simulink model "RL_tcp_2021b"  (R2021b)
settings: Solver=VariableStepAuto  StartTime=0.0  StopTime=inf  RelTol=1e-3
undefined symbols (not defined in the file or in its folder): A, alpha_b_gain, B, C, Discrete, fitresultpowertwoFL, fitresultpowertwoFR, fitresultpowertwoRL, fitresultpowertwoRR, R, rotateCorrectionCoef, Tf, Time, Ts, VRef, x_norm_min, y_norm_min, y_norm_range, z_l_gain
libraries: svdutilitieslib x15, simulink x9, ctrlSharedLib x3, instrumentlib x2, deeplib x2, aerolibanimutils x1
settings Model: Creator=4DLab5  LastModifiedBy=n7729

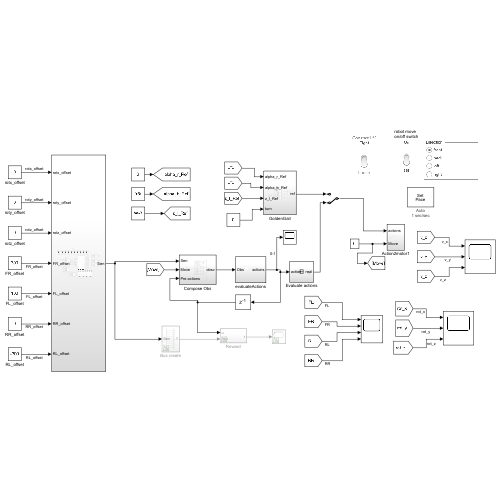
[thumbnail: Simulink's stored preview of the top-level diagram]
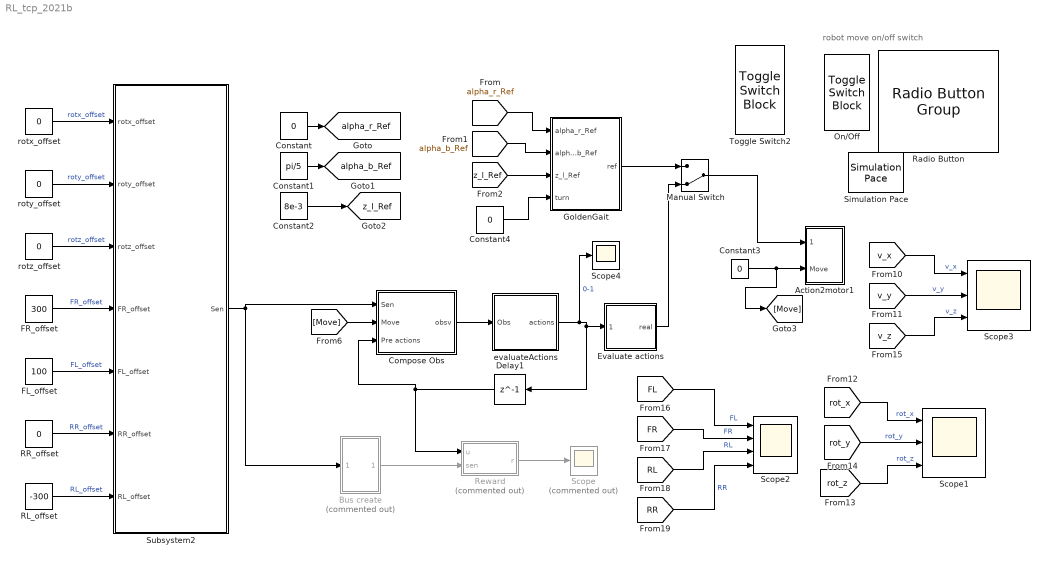
== system RL_tcp_2021b ==
  note: robot move
      | on/off switch
  Action2motor1 : Subsystem
  Bus create : Subsystem  Commented=on
  Compose Obs : Subsystem
  Constant : Constant  Value=0
  Constant1 : Constant  Value=pi/5
  Constant2 : Constant  Value=8e-3
  Constant3 : Constant  Value=0
  Constant4 : Constant  Value=0
  Delay1 : Delay  DelayLength=1  InitialCondition=[0.5;0.5;0.5;0.5]  SampleTime=0.05
  Evaluate actions : Subsystem
  FL_offset : Constant  Value=100
  FR_offset : Constant  Value=300
  GoldenGait : Subsystem
  Manual Switch : ManualSwitch  CurrentSetting=0
  On/Off : ToggleSwitchBlock  LabelPosition=Hide
      settings: Values={{'Off', 'On'}, [0 1]}
  RL_offset : Constant  Value=-300
  RR_offset : Constant  Value=0
  Radio Button : RadioButtonGroup  LabelPosition=Hide  SelectedLabel=front  ButtonGroupName=Direction
      settings: Values={{'front', 'back', 'left', 'right'}, [0 3.1416 1.5708 -1.5708]}
  Reward : Subsystem  Commented=on
  Scope : Scope  Commented=on
  Scope1 : Scope  NumInputPorts=3
  Scope2 : Scope  NumInputPorts=4
  Scope3 : Scope  NumInputPorts=3
  Scope4 : Scope
  Simulation Pace : aerolibanimutils/Simulation Pace  SimulationPace=1  SleepMode=Auto  OutputPaceError=off  SampleTime=0.05
  Subsystem2 : Subsystem
  Toggle Switch2 : ToggleSwitchBlock
      settings: Values={{'Loose', 'Tight'}, [0 1]}
  evaluateActions : Subsystem
  rotx_offset : Constant  Value=0
  roty_offset : Constant  Value=0
  rotz_offset : Constant  Value=0
  tag scope: alpha_b_Ref=global, alpha_r_Ref=global, z_l_Ref=global
  wires:
  RR_offset/1 -> Subsystem2/6(RR_offset)  "RR_offset"
  [v_x] -> Scope3/1  "v_x"
  RL_offset/1 -> Subsystem2/7(RL_offset)  "RL_offset"
  [Move] -> Compose Obs/2(Move)
  [rot_y] -> Scope1/2  "rot_y"
  Evaluate actions/1(real) -> Manual Switch/2
  FR_offset/1 -> Subsystem2/4(FR_offset)  "FR_offset"
  [RL] -> Scope2/3  "RL"
  [rot_z] -> Scope1/3  "rot_z"
  Constant4/1 -> GoldenGait/4(turn)
  [RR] -> Scope2/4  "RR"
  [alpha_r_Ref] -> GoldenGait/1(alpha_r_Ref)
  Delay1/1 -> Compose Obs/3(Pre actions), Reward/1(u)
  [z_l_Ref] -> GoldenGait/3(z_l_Ref)
  [v_z] -> Scope3/3  "v_z"
  [v_y] -> Scope3/2  "v_y"
  [FR] -> Scope2/2  "FR"
  [alpha_b_Ref] -> GoldenGait/2(alpha_b_Ref)
  [rot_x] -> Scope1/1  "rot_x"
  Manual Switch/1 -> Action2motor1/1(actions)
  [FL] -> Scope2/1  "FL"
  Subsystem2/1(Sen) -> Compose Obs/1(Sen), Bus create/1(Sen)
  Compose Obs/1(obsv) -> evaluateActions/1(Obs)
  Constant1/1 -> [alpha_b_Ref]
  Constant2/1 -> [z_l_Ref]
  Constant3/1 -> [Move], Action2motor1/2(Move)
  rotz_offset/1 -> Subsystem2/3(rotz_offset)  "rotz_offset"
  roty_offset/1 -> Subsystem2/2(roty_offset)  "roty_offset"
  Reward/1(r) -> Scope/1
  Constant/1 -> [alpha_r_Ref]
  Bus create/1(Outport) -> Reward/2(sen)
  FL_offset/1 -> Subsystem2/5(FL_offset)  "FL_offset"
  evaluateActions/1(actions) -> Scope4/1, Evaluate actions/1(action), Delay1/1  "0-1"
  GoldenGait/1(ref) -> Manual Switch/1
  rotx_offset/1 -> Subsystem2/1(rotx_offset)  "rotx_offset"

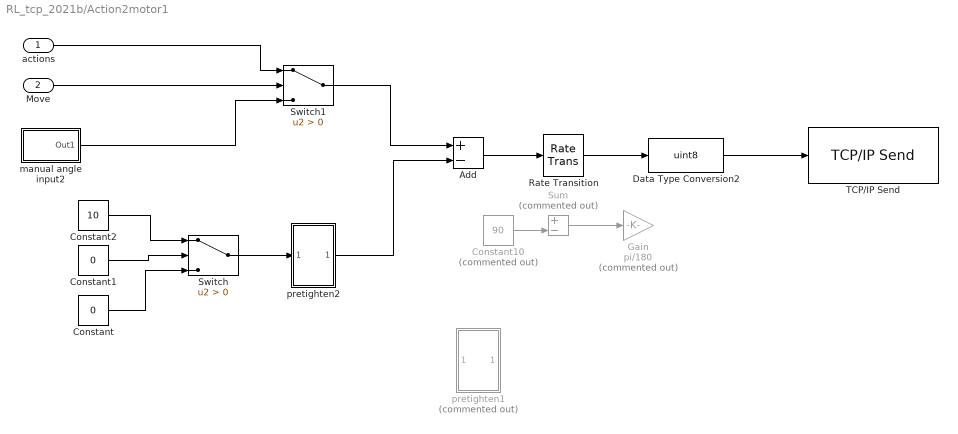
== system RL_tcp_2021b/Action2motor1 ==
  actions : Inport
  Move : Inport  Port=2
  Add : Sum  Inputs=+-
  Constant : Constant  Value=0
  Constant1 : Constant  Value=0
  Constant10 : Constant  Commented=on  Value=90
  Constant2 : Constant  Value=10
  Data Type Conversion2 : DataTypeConversion  OutDataTypeStr=uint8
  Gain : Gain  Commented=on  Gain=pi/180
  Rate Transition : RateTransition  OutPortSampleTime=0.05
  Sum : Sum  Commented=on  Inputs=+-
  Switch : Switch  Criteria=u2 > Threshold
  Switch1 : Switch  Criteria=u2 > Threshold
  TCP/IP Send : instrumentlib/TCP//IP Send  Priority=1  Host=192.168.0.103  Port=6666  ByteOrder=big-endian  EnableBlockingMode=on  Timeout=1  TransferDelay=on  SimulateUsing=Interpreted execution
  manual angle input2 : Subsystem
  pretighten1 : Subsystem  Commented=on
  pretighten2 : Subsystem
  wires:
  manual angle input2/1(Out1) -> Switch1/3
  pretighten2/1(Out1) -> Add/2
  Switch1/1 -> Add/1
  Switch/1 -> pretighten2/1(In1)
  Constant/1 -> Switch/3
  Constant2/1 -> Switch/1
  Data Type Conversion2/1 -> TCP/IP Send/1
  Add/1 -> Rate Transition/1
  Constant1/1 -> Switch/2
  Move/1 -> Switch1/2
  actions/1 -> Switch1/1
  Constant10/1 -> Sum/2
  Sum/1 -> Gain/1
  Rate Transition/1 -> Data Type Conversion2/1

== system RL_tcp_2021b/Bus create ==
  Sen : Inport
  Bus Creator : BusCreator  Inputs=10
  Demux : Demux  Outputs=10
  Outport : Outport
  wires:
  Sen/1 -> Demux/1
  Demux/1 -> Bus Creator/1  "rot_x"
  Demux/2 -> Bus Creator/2  "rot_y"
  Demux/3 -> Bus Creator/3  "rot_z"
  Bus Creator/1 -> Outport/1
  Demux/4 -> Bus Creator/4  "v_x"
  Demux/5 -> Bus Creator/5  "v_y"
  Demux/6 -> Bus Creator/6  "v_z"
  Demux/7 -> Bus Creator/7  "FnFR"
  Demux/8 -> Bus Creator/8  "FnFL"
  Demux/9 -> Bus Creator/9  "FnRL"
  Demux/10 -> Bus Creator/10  "FnRR"

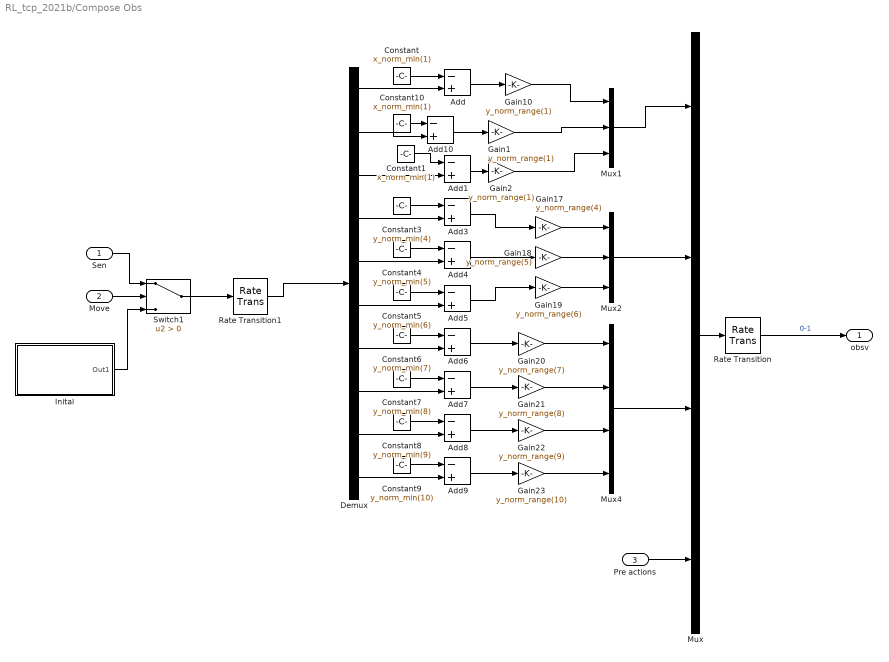
== system RL_tcp_2021b/Compose Obs ==
  Sen : Inport
  Move : Inport  Port=2
  Pre actions : Inport  Port=3
  Add{,1,3..10} (10 alike) : Sum  Inputs=-+
  Constant : Constant  Value=x_norm_min(1)
  Constant1 : Constant  Value=x_norm_min(1)
  Constant10 : Constant  Value=x_norm_min(1)
  Constant3 : Constant  Value=y_norm_min(4)
  Constant4 : Constant  Value=y_norm_min(5)
  Constant5 : Constant  Value=y_norm_min(6)
  Constant6 : Constant  Value=y_norm_min(7)
  Constant7 : Constant  Value=y_norm_min(8)
  Constant8 : Constant  Value=y_norm_min(9)
  Constant9 : Constant  Value=y_norm_min(10)
  Demux : Demux  Outputs=10
  Gain1 : Gain  Gain=y_norm_range(1)
  Gain10 : Gain  Gain=y_norm_range(1)
  Gain17 : Gain  Gain=y_norm_range(4)
  Gain18 : Gain  Gain=y_norm_range(5)
  Gain19 : Gain  Gain=y_norm_range(6)
  Gain2 : Gain  Gain=y_norm_range(1)
  Gain20 : Gain  Gain=y_norm_range(7)
  Gain21 : Gain  Gain=y_norm_range(8)
  Gain22 : Gain  Gain=y_norm_range(9)
  Gain23 : Gain  Gain=y_norm_range(10)
  Inital : Subsystem
  Mux : Mux
  Mux1 : Mux  Inputs=3
  Mux2 : Mux  Inputs=3
  Mux4 : Mux
  Rate Transition : RateTransition  OutPortSampleTime=Ts
  Rate Transition1 : RateTransition  OutPortSampleTime=Ts
  Switch1 : Switch  Criteria=u2 > Threshold
  obsv : Outport  VectorParamsAs1DForOutWhenUnconnected=off
  wires:
  Gain18/1 -> Mux2/2
  Gain19/1 -> Mux2/3
  Constant/1 -> Add/1
  Gain10/1 -> Mux1/1
  Add/1 -> Gain10/1
  Mux2/1 -> Mux/2
  Constant5/1 -> Add5/1
  Demux/1 -> Add/2
  Gain21/1 -> Mux4/2
  Demux/9 -> Add8/2
  Add9/1 -> Gain23/1
  Constant9/1 -> Add9/1
  Rate Transition/1 -> obsv/1  "0-1"
  Add3/1 -> Gain17/1
  Constant7/1 -> Add7/1
  Gain20/1 -> Mux4/1
  Gain17/1 -> Mux2/1
  Constant6/1 -> Add6/1
  Demux/4 -> Add3/2
  Mux4/1 -> Mux/3
  Mux/1 -> Rate Transition/1
  Add7/1 -> Gain21/1
  Mux1/1 -> Mux/1
  Demux/7 -> Add6/2
  Gain23/1 -> Mux4/4
  Demux/5 -> Add4/2
  Gain22/1 -> Mux4/3
  Constant4/1 -> Add4/1
  Constant3/1 -> Add3/1
  Constant8/1 -> Add8/1
  Add5/1 -> Gain19/1
  Add4/1 -> Gain18/1
  Add6/1 -> Gain20/1
  Add8/1 -> Gain22/1
  Demux/8 -> Add7/2
  Pre actions/1 -> Mux/4
  Demux/10 -> Add9/2
  Demux/6 -> Add5/2
  Move/1 -> Switch1/2
  Sen/1 -> Switch1/1
  Switch1/1 -> Rate Transition1/1
  Inital/1(Out1) -> Switch1/3
  Rate Transition1/1 -> Demux/1
  Demux/2 -> Add10/2
  Add10/1 -> Gain1/1
  Gain1/1 -> Mux1/2
  Constant10/1 -> Add10/1
  Add1/1 -> Gain2/1
  Demux/3 -> Add1/2
  Gain2/1 -> Mux1/3
  Constant1/1 -> Add1/1

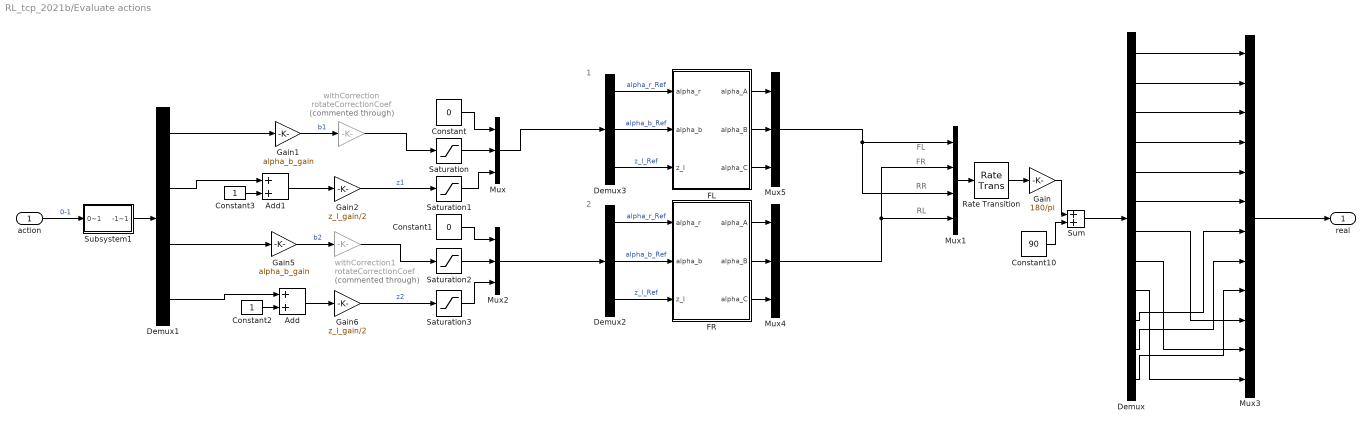
== system RL_tcp_2021b/Evaluate actions ==
  note: RL
  note: FR
  note: FL
  note: RR
  note: 2
  note: 1
  action : Inport
  Add : Sum
  Add1 : Sum
  Constant : Constant  Value=0
  Constant1 : Constant  Value=0
  Constant10 : Constant  Value=90
  Constant2 : Constant
  Constant3 : Constant
  Demux : Demux  Outputs=12
  Demux1 : Demux
  Demux2 : Demux  Outputs=3
  Demux3 : Demux  Outputs=3
  FL : MATLAB Function  TreatAsAtomicUnit=on
  FR : MATLAB Function  TreatAsAtomicUnit=on
  Gain : Gain  Gain=180/pi
  Gain1 : Gain  Gain=alpha_b_gain
  Gain2 : Gain  Gain=z_l_gain/2
  Gain5 : Gain  Gain=alpha_b_gain
  Gain6 : Gain  Gain=z_l_gain/2
  Mux{,2,4..5} (4 alike) : Mux  Inputs=3
  Mux1 : Mux
  Mux3 : Mux  Inputs=12
  Rate Transition : RateTransition  OutPortSampleTime=0.05
  Saturation : Saturate  UpperLimit=pi/5  LowerLimit=-pi/5
  Saturation1 : Saturate  UpperLimit=10e-3  LowerLimit=-10e-3
  Saturation2 : Saturate  UpperLimit=pi/5  LowerLimit=-pi/5
  Saturation3 : Saturate  UpperLimit=10e-3  LowerLimit=-10e-3
  Subsystem1 : Subsystem
  Sum : Sum
  withCorrection : Gain  Commented=through  Gain=rotateCorrectionCoef
  withCorrection1 : Gain  Commented=through  Gain=rotateCorrectionCoef
  real : Outport
  wires:
  Mux1/1 -> Rate Transition/1
  Constant/1 -> Mux/1
  withCorrection/1 -> Saturation/1
  Constant1/1 -> Mux2/1
  withCorrection1/1 -> Saturation2/1
  Mux2/1 -> Demux2/1
  Saturation/1 -> Mux/2
  Saturation2/1 -> Mux2/2
  Saturation1/1 -> Mux/3
  Saturation3/1 -> Mux2/3
  action/1 -> Subsystem1/1(0~1)  "0-1"
  Demux1/1 -> Gain1/1
  Gain1/1 -> withCorrection/1  "b1"
  Gain5/1 -> withCorrection1/1  "b2"
  Gain2/1 -> Saturation1/1  "z1"
  Gain6/1 -> Saturation3/1  "z2"
  Demux1/2 -> Add1/1
  Add1/1 -> Gain2/1
  Add/1 -> Gain6/1
  Constant2/1 -> Add/2
  Demux1/3 -> Gain5/1
  Constant3/1 -> Add1/2
  Demux1/4 -> Add/1
  Subsystem1/1(-1~1) -> Demux1/1
  Sum/1 -> Demux/1
  Demux/11 -> Mux3/8
  Gain/1 -> Sum/1
  Demux/2 -> Mux3/2
  Demux/10 -> Mux3/7
  Demux/9 -> Mux3/12
  Demux/5 -> Mux3/5
  Demux/1 -> Mux3/1
  Demux/7 -> Mux3/10
  Demux/8 -> Mux3/11
  Demux/4 -> Mux3/4
  Demux/12 -> Mux3/9
  Constant10/1 -> Sum/2
  Demux/6 -> Mux3/6
  Demux/3 -> Mux3/3
  Demux2/1 -> FR/1(alpha_r)  "alpha_r_Ref"
  FR/3(alpha_C) -> Mux4/3
  Demux2/2 -> FR/2(alpha_b)  "alpha_b_Ref"
  FR/2(alpha_B) -> Mux4/2
  FR/1(alpha_A) -> Mux4/1
  Mux4/1 -> Mux1/2, Mux1/4
  Demux2/3 -> FR/3(z_l)  "z_l_Ref"
  Mux3/1 -> real/1
  FL/1(alpha_A) -> Mux5/1
  Mux5/1 -> Mux1/3, Mux1/1
  Demux3/3 -> FL/3(z_l)  "z_l_Ref"
  FL/3(alpha_C) -> Mux5/3
  FL/2(alpha_B) -> Mux5/2
  Mux/1 -> Demux3/1
  Demux3/1 -> FL/1(alpha_r)  "alpha_r_Ref"
  Demux3/2 -> FL/2(alpha_b)  "alpha_b_Ref"
  Rate Transition/1 -> Gain/1

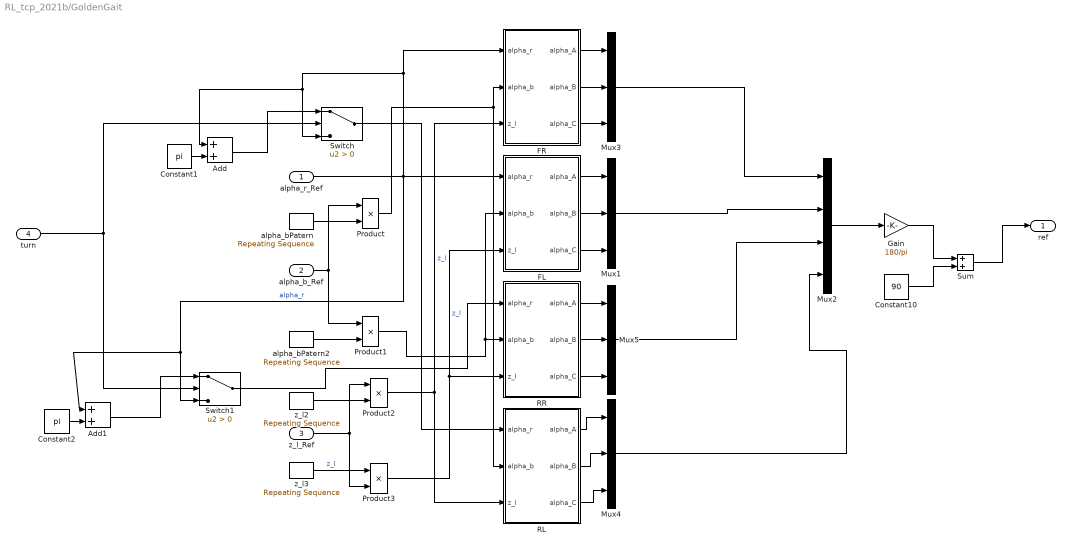
== system RL_tcp_2021b/GoldenGait ==
  alpha_r_Ref : Inport
  alpha_b_Ref : Inport  Port=2
  z_l_Ref : Inport  Port=3
  turn : Inport  Port=4
  Add : Sum
  Add1 : Sum
  Constant1 : Constant  Value=pi
  Constant10 : Constant  Value=90
  Constant2 : Constant  Value=pi
  FL : MATLAB Function  TreatAsAtomicUnit=on
  FR : MATLAB Function  TreatAsAtomicUnit=on
  Gain : Gain  Gain=180/pi
  Mux{1,3..5} (4 alike) : Mux  Inputs=3
  Mux2 : Mux
  Product{,1..3} (4 alike) : Product
  RL : MATLAB Function  TreatAsAtomicUnit=on
  RR : MATLAB Function  TreatAsAtomicUnit=on
  Sum : Sum
  Switch : Switch  Criteria=u2 > Threshold
  Switch1 : Switch  Criteria=u2 > Threshold
  alpha_bPatern : simulink/Sources/Repeating Sequence  rep_seq_t=[0 0.2 0.4 0.6 0.8]  rep_seq_y=[0 1 0 -1 0]
  alpha_bPatern2 : simulink/Sources/Repeating Sequence  rep_seq_t=[0 0.2 0.4 0.6 0.8]  rep_seq_y=[0 -1 0 1 0]
  z_l2 : simulink/Sources/Repeating Sequence  rep_seq_t=[0 0.2 0.4 0.6 0.8]  rep_seq_y=[0 1 1 1 0]
  z_l3 : simulink/Sources/Repeating Sequence  rep_seq_t=[0 0.2 0.4 0.6 0.8]  rep_seq_y=[1 1 0 1 1]
  ref : Outport
  wires:
  FR/1(alpha_A) -> Mux3/1
  Product2/1 -> FR/3(z_l), RL/3(z_l)  "z_l"
  FR/2(alpha_B) -> Mux3/2
  FR/3(alpha_C) -> Mux3/3
  Product3/1 -> FL/3(z_l), RR/3(z_l)  "z_l"
  FL/3(alpha_C) -> Mux1/3
  alpha_r_Ref/1 -> Switch1/3, Add1/1, FL/1(alpha_r), FR/1(alpha_r), Switch/3, Add/1  "alpha_r"
  FL/2(alpha_B) -> Mux1/2
  FL/1(alpha_A) -> Mux1/1
  alpha_bPatern/1 -> Product/2
  alpha_b_Ref/1 -> Product/1, Product1/1
  Product/1 -> RL/2(alpha_b), FR/2(alpha_b)
  alpha_bPatern2/1 -> Product1/2
  Product1/1 -> FL/2(alpha_b), RR/2(alpha_b)
  z_l2/1 -> Product2/2
  z_l_Ref/1 -> Product3/2, Product2/1
  z_l3/1 -> Product3/1  "z_l"
  RL/3(alpha_C) -> Mux4/3
  RL/2(alpha_B) -> Mux4/2
  RL/1(alpha_A) -> Mux4/1
  Mux3/1 -> Mux2/1
  RR/3(alpha_C) -> Mux5/3
  RR/1(alpha_A) -> Mux5/1
  RR/2(alpha_B) -> Mux5/2
  Switch/1 -> RL/1(alpha_r)
  Constant1/1 -> Add/2
  Add/1 -> Switch/1
  Switch1/1 -> RR/1(alpha_r)
  Add1/1 -> Switch1/1
  Constant2/1 -> Add1/2
  turn/1 -> Switch1/2, Switch/2
  Mux1/1 -> Mux2/2
  Mux4/1 -> Mux2/4
  Mux5/1 -> Mux2/3
  Sum/1 -> ref/1
  Mux2/1 -> Gain/1
  Constant10/1 -> Sum/2
  Gain/1 -> Sum/1

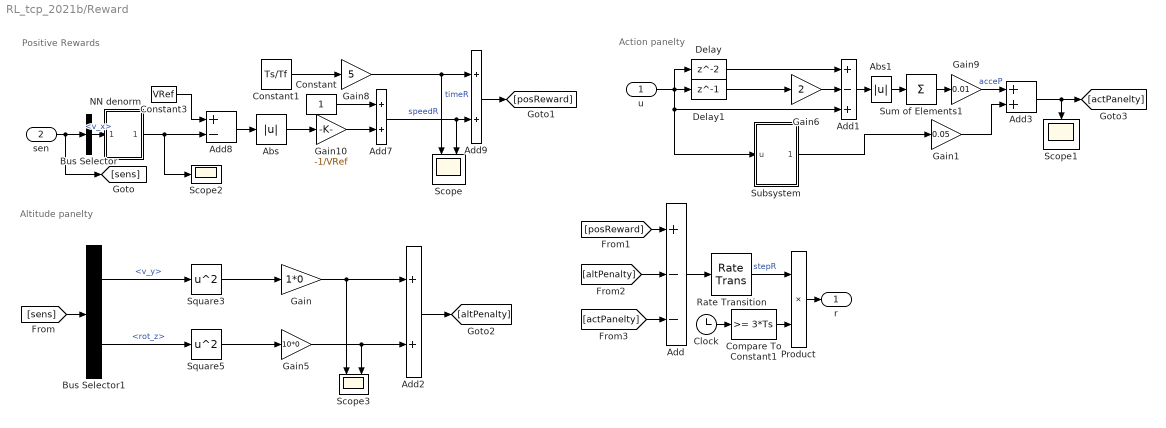
== system RL_tcp_2021b/Reward ==
  note: Action panelty
  note: Altitude panelty
  note: Positive Rewards
  u : Inport
  sen : Inport  Port=2
  Abs : Abs
  Abs1 : Abs
  Add : Sum  Inputs=+--
  Add1 : Sum  Inputs=+-+
  Add{2..3,7,9} (4 alike) : Sum
  Add8 : Sum  Inputs=+-
  Bus Selector : BusSelector  OutputSignals=v_x
  Bus Selector1 : BusSelector  OutputSignals=v_y,rot_z
  Clock : Clock
  Compare To Constant1 : simulink/Logic and Bit Operations/Compare To Constant  relop=>=  const=3*Ts  OutDataTypeStr=boolean
  Constant : Constant
  Constant1 : Constant  Value=Ts/Tf
  Constant3 : Constant  Value=VRef
  Delay : Delay  InitialCondition=0.5
  Delay1 : Delay  DelayLength=1  InitialCondition=0.5
  Gain : Gain  Gain=1*0
  Gain1 : Gain  Gain=0.05
  Gain10 : Gain  Gain=-1/VRef
  Gain5 : Gain  Gain=10*0
  Gain6 : Gain  Gain=2
  Gain8 : Gain  Gain=5
  Gain9 : Gain  Gain=0.01
  NN denorm : Subsystem
  Product : Product
  Rate Transition : RateTransition  OutPortSampleTime=Ts
  Scope : Scope  NumInputPorts=2
  Scope1 : Scope
  Scope2 : Scope
  Scope3 : Scope  NumInputPorts=2
  Square3 : Math  Operator=square  SignedPower=on  SaturateOnIntegerOverflow=on
  Square5 : Math  Operator=square  SignedPower=on  SaturateOnIntegerOverflow=on
  Subsystem : Subsystem
  Sum of Elements1 : Sum  Inputs=+
  r : Outport  VectorParamsAs1DForOutWhenUnconnected=off
  wires:
  sen/1 -> Bus Selector/1, [sens]
  Square3/1 -> Gain/1
  Square5/1 -> Gain5/1
  Bus Selector1/2 -> Square5/1  "<rot_z>"
  Gain/1 -> Scope3/1, Add2/1
  Add/1 -> Rate Transition/1
  Constant1/1 -> Gain8/1
  Delay/1 -> Add1/1
  Gain6/1 -> Add1/2
  Add1/1 -> Abs1/1
  Abs1/1 -> Sum of Elements1/1
  Delay1/1 -> Gain6/1
  u/1 -> Subsystem/1(u), Add1/3, Delay/1, Delay1/1
  Sum of Elements1/1 -> Gain9/1
  Clock/1 -> Compare To Constant1/1
  Compare To Constant1/1 -> Product/2
  Rate Transition/1 -> Product/1  "stepR"
  Product/1 -> r/1
  [sens] -> Bus Selector1/1
  Gain8/1 -> Add9/1, Scope/1  "timeR"
  Add9/1 -> [posReward]
  Bus Selector1/1 -> Square3/1  "<v_y>"
  Gain5/1 -> Add2/2, Scope3/2
  Add2/1 -> [altPenalty]
  [posReward] -> Add/1
  [altPenalty] -> Add/2
  [actPanelty] -> Add/3
  Add8/1 -> Abs/1
  Add7/1 -> Scope/2, Add9/2  "speedR"
  Gain10/1 -> Add7/2
  Abs/1 -> Gain10/1
  Constant/1 -> Add7/1
  Constant3/1 -> Add8/1
  Bus Selector/1 -> NN denorm/1(In1)  "<v_x>"
  NN denorm/1(Out1) -> Scope2/1, Add8/2
  Gain9/1 -> Add3/1  "acceP"
  Add3/1 -> Scope1/1, [actPanelty]
  Subsystem/1(Out1) -> Gain1/1
  Gain1/1 -> Add3/2

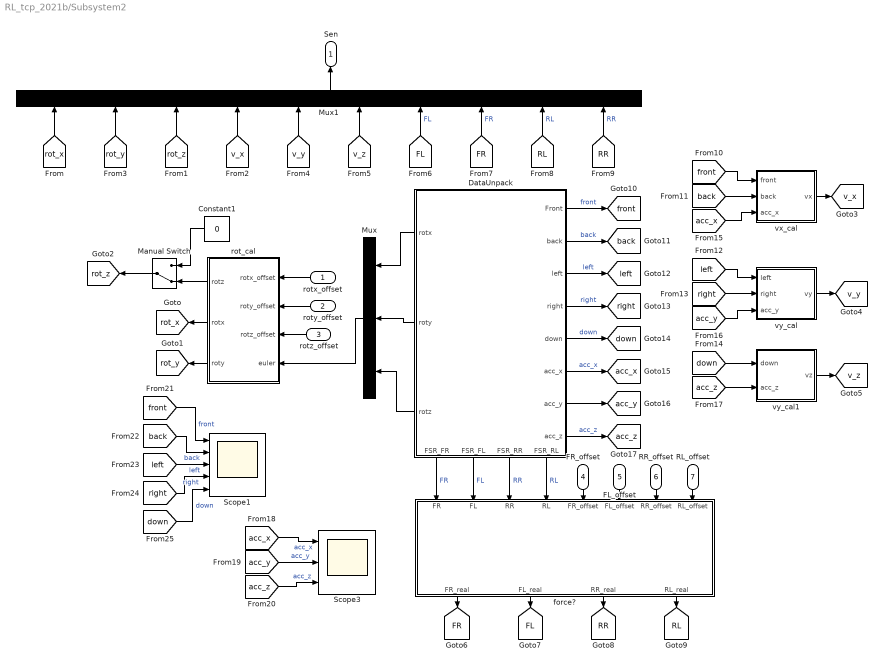
== system RL_tcp_2021b/Subsystem2 ==
  rotx_offset : Inport
  roty_offset : Inport  Port=2
  rotz_offset : Inport  Port=3
  FR_offset : Inport  Port=4
  FL_offset : Inport  Port=5
  RR_offset : Inport  Port=6
  RL_offset : Inport  Port=7
  Constant1 : Constant  Value=0
  DataUnpack : Subsystem
      settings: PortSchema="{\"entries\":[{\"content\":{\"sides\":[{\"content\":{\"connectorIds\":[\"Out13\",\"Out14\",\"Out15\"]},\"type\":\"ConnectorPlacement.EquallySpacedRectSide\",\"uuid\":\"921b036b-a103-4c29-98a4-1e13be366f27\"},{\"content\":{\"connectorIds\":[\"Out1\",\"Out2\",\"Out3\",\"Out4\",\"Out5\",\"Out6\",\"Out7\",\"Out8\"],\"side\":\"RIGHT\"},\"type\":\"ConnectorPlacement.EquallySpacedRectSide\",\"uuid\":\"743cc973-2ca6-4eb4-ab94-a827ba3cd866\"},{\"content\":{\"side\":\"TOP\"},\"type\":\"ConnectorPlacement.EquallySpacedRectSide\",\"uuid\":\"9eb642df-d260-4317-8a72-bd8569bebf98\"},{\"content\":{\"connectorIds\":[\"Out9\",\"Out10\",\"Out11\",\"Out12\"],\"side\":\"BOTTOM\"},\"type\":\"ConnectorPlacement.EquallySpacedRectSide\",\"uuid\":\"da7ab237-c829-42b0-bbc7-f99a364eb64c\"}]},\"type\":\"ConnectorPlacement.EquallySpacedConnector\",\"uuid\":\"aa8a793e-4baf-4a67-be1f-284a705b408b\"}],\"packageUris\":[\"http://schema.mathworks.com/mf0/Connector/R2020b\"],\"version\":\"1.0\"}"
  Manual Switch : ManualSwitch  CurrentSetting=0
  Mux : Mux  Inputs=3
  Mux1 : Mux  Inputs=10
  Scope1 : Scope  NumInputPorts=5
  Scope3 : Scope  NumInputPorts=3
  force? : Subsystem
  rot_cal : Subsystem
  vx_cal : Subsystem
  vy_cal : Subsystem
  vy_cal1 : Subsystem
  Sen : Outport
  tag scope: FL=global, FR=global, RL=global, RR=global, acc_x=global, acc_y=global, acc_z=global, back=global, down=global, front=global, left=global, right=global, rot_x=global, rot_y=global, rot_z=global, v_x=global, v_y=global, v_z=global
  wires:
  rotz_offset/1 -> rot_cal/3(rotz_offset)
  DataUnpack/14(roty) -> Mux/2
  RL_offset/1 -> force?/8(RL_offset)
  Mux/1 -> rot_cal/4(euler)
  DataUnpack/13(rotx) -> Mux/1
  FL_offset/1 -> force?/6(FL_offset)
  FR_offset/1 -> force?/5(FR_offset)
  DataUnpack/15(rotz) -> Mux/3
  RR_offset/1 -> force?/7(RR_offset)
  roty_offset/1 -> rot_cal/2(roty_offset)
  rotx_offset/1 -> rot_cal/1(rotx_offset)
  force?/1(FR_real) -> [FR]
  force?/2(FL_real) -> [FL]
  force?/3(RR_real) -> [RR]
  force?/4(RL_real) -> [RL]
  vx_cal/1(vx) -> [v_x]
  vy_cal/1(vy) -> [v_y]
  vy_cal1/1(vz) -> [v_z]
  rot_cal/2(rotx) -> [rot_x]
  rot_cal/3(roty) -> [rot_y]
  Manual Switch/1 -> [rot_z]
  DataUnpack/9(FSR_FR) -> force?/1(FR)  "FR"
  DataUnpack/10(FSR_FL) -> force?/2(FL)  "FL"
  DataUnpack/11(FSR_RR) -> force?/3(RR)  "RR"
  DataUnpack/12(FSR_RL) -> force?/4(RL)  "RL"
  [rot_x] -> Mux1/1
  [rot_y] -> Mux1/2
  [rot_z] -> Mux1/3
  [v_x] -> Mux1/4
  [v_y] -> Mux1/5
  [v_z] -> Mux1/6
  [FL] -> Mux1/7  "FL"
  [FR] -> Mux1/8  "FR"
  [RL] -> Mux1/9  "RL"
  [RR] -> Mux1/10  "RR"
  Mux1/1 -> Sen/1
  Constant1/1 -> Manual Switch/1
  rot_cal/1(rotz) -> Manual Switch/2
  [acc_z] -> Scope3/3  "acc_z"
  [acc_y] -> Scope3/2  "acc_y"
  [acc_x] -> Scope3/1  "acc_x"
  DataUnpack/1(Front) -> [front]  "front"
  DataUnpack/2(back) -> [back]  "back"
  DataUnpack/3(left) -> [left]  "left"
  DataUnpack/4(right) -> [right]  "right"
  DataUnpack/5(down) -> [down]  "down"
  [front] -> vx_cal/1(front)
  [back] -> vx_cal/2(back)
  DataUnpack/6(acc_x) -> [acc_x]  "acc_x"
  DataUnpack/7(acc_y) -> [acc_y]
  DataUnpack/8(acc_z) -> [acc_z]  "acc_z"
  [left] -> vy_cal/1(left)
  [right] -> vy_cal/2(right)
  [down] -> vy_cal1/1(down)
  [acc_x] -> vx_cal/3(acc_x)
  [acc_y] -> vy_cal/3(acc_y)
  [acc_z] -> vy_cal1/2(acc_z)
  [front] -> Scope1/1  "front"
  [back] -> Scope1/2  "back"
  [left] -> Scope1/3  "left"
  [right] -> Scope1/4  "right"
  [down] -> Scope1/5  "down"

== system RL_tcp_2021b/evaluateActions ==
  Obs : Inport
  Cast To Double : DataTypeConversion  OutDataTypeStr=double
  MATLAB Function1 : MATLAB Function  TreatAsAtomicUnit=on
  MATLAB Function2 : MATLAB Function  Commented=on  TreatAsAtomicUnit=on
  Predict : deeplib/Predict  Commented=on  Network=Network from MAT-file  NetworkFunction=squeezenet  NetworkFilePath=C:\Users\4DLab5\Desktop\Xuezhi\real_robot\Agent606home.mat  MiniBatchSize=128  InputDataFormats={ 'observation', '[1x22]' }  Predictions=on  Activations={}  ForceInterpretedSim=off  EnableDLNetwork=on
      settings: SourceProductBaseCode=NN
  Predict2 : deeplib/Predict  Network=Network from MAT-file  NetworkFunction=evaluatePolicy  NetworkFilePath=D:\KTH-MasterThesis\Simulink_models\agentData.mat  MiniBatchSize=256  InputDataFormats={ 'observation', '' }  Predictions=on  Activations={}  ForceInterpretedSim=off  EnableDLNetwork=on
      settings: SourceProductBaseCode=NN
  Rate Transition : RateTransition  Commented=through  OutPortSampleTime=0.05
  Transpose : Math  Operator=transpose  SaturateOnIntegerOverflow=on
  Transpose1 : Math  Operator=transpose  SaturateOnIntegerOverflow=on
  Zero-Order Hold : ZeroOrderHold  Commented=through  SampleTime=0.1
  actions : Outport  OutDataTypeStr=double
  wires:
  Cast To Double/1 -> Transpose1/1
  Obs/1 -> Transpose/1
  Rate Transition/1 -> Cast To Double/1
  Predict2/1 -> Rate Transition/1  "meanAndStd"
  Transpose1/1 -> MATLAB Function1/1(meanAndStd)
  MATLAB Function1/1(action1) -> actions/1
  Zero-Order Hold/1 -> Predict2/1
  Transpose/1 -> Zero-Order Hold/1

== system RL_tcp_2021b/Action2motor1/manual angle input2 ==
  Constant{,3..13} (12 alike) : Constant  Value=90  SampleTime=-1
  Mux : Mux  Inputs=12
  Out1 : Outport
  wires:
  Constant3/1 -> Mux/2
  Constant11/1 -> Mux/10
  Constant9/1 -> Mux/8
  Constant8/1 -> Mux/7
  Constant/1 -> Mux/1
  Constant4/1 -> Mux/3
  Constant10/1 -> Mux/9
  Constant5/1 -> Mux/4
  Constant7/1 -> Mux/6
  Constant13/1 -> Mux/12
  Constant12/1 -> Mux/11
  Constant6/1 -> Mux/5
  Mux/1 -> Out1/1

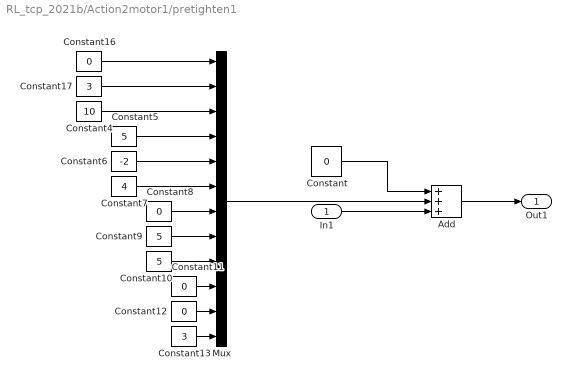
== system RL_tcp_2021b/Action2motor1/pretighten1 ==
  In1 : Inport
  Add : Sum  Inputs=+++
  Constant : Constant  Value=0
  Constant10 : Constant  Value=5  SampleTime=-1
  Constant{8,11..12,16} (4 alike) : Constant  Value=0  SampleTime=-1
  Constant13 : Constant  Value=3  SampleTime=-1
  Constant17 : Constant  Value=3  SampleTime=-1
  Constant4 : Constant  Value=10  SampleTime=-1
  Constant5 : Constant  Value=5  SampleTime=-1
  Constant6 : Constant  Value=-2  SampleTime=-1
  Constant7 : Constant  Value=4  SampleTime=-1
  Constant9 : Constant  Value=5  SampleTime=-1
  Mux : Mux  Inputs=12
  Out1 : Outport
  wires:
  Constant12/1 -> Mux/11
  Constant6/1 -> Mux/5
  Constant9/1 -> Mux/8
  Constant4/1 -> Mux/3
  Constant13/1 -> Mux/12
  Constant7/1 -> Mux/6
  Constant5/1 -> Mux/4
  Mux/1 -> Add/2
  Constant10/1 -> Mux/9
  Constant8/1 -> Mux/7
  Constant11/1 -> Mux/10
  Constant17/1 -> Mux/2
  Constant/1 -> Add/1
  Constant16/1 -> Mux/1
  Add/1 -> Out1/1
  In1/1 -> Add/3

== system RL_tcp_2021b/Action2motor1/pretighten2 ==
  In1 : Inport
  Add : Sum  Inputs=+++
  Constant : Constant  Value=0
  Constant10 : Constant  Value=9  SampleTime=-1
  Constant11 : Constant  Value=4  SampleTime=-1
  Constant12 : Constant  Value=0  SampleTime=-1
  Constant13 : Constant  Value=10  SampleTime=-1
  Constant16 : Constant  SampleTime=-1
  Constant17 : Constant  Value=8  SampleTime=-1
  Constant4 : Constant  Value=10  SampleTime=-1
  Constant5 : Constant  Value=-7  SampleTime=-1
  Constant6 : Constant  Value=-3  SampleTime=-1
  Constant7 : Constant  Value=5  SampleTime=-1
  Constant8 : Constant  Value=-2  SampleTime=-1
  Constant9 : Constant  Value=12  SampleTime=-1
  Mux : Mux  Inputs=12
  Out1 : Outport
  wires:
  Constant12/1 -> Mux/11
  Constant6/1 -> Mux/5
  Constant9/1 -> Mux/8
  Constant4/1 -> Mux/3
  Constant13/1 -> Mux/12
  Constant7/1 -> Mux/6
  Constant5/1 -> Mux/4
  Mux/1 -> Add/2
  Constant10/1 -> Mux/9
  Constant8/1 -> Mux/7
  Constant11/1 -> Mux/10
  Constant17/1 -> Mux/2
  Constant/1 -> Add/1
  Constant16/1 -> Mux/1
  Add/1 -> Out1/1
  In1/1 -> Add/3

== system RL_tcp_2021b/Compose Obs/Inital ==
  Constant{10..15} (6 alike) : Constant  Value=0
  Constant{16..19} (4 alike) : Constant  Value=5
  Mux3 : Mux  Inputs=10
  Out1 : Outport
  wires:
  Constant19/1 -> Mux3/10  "RR"
  Constant12/1 -> Mux3/3  "rotz"
  Constant11/1 -> Mux3/2  "roty"
  Constant14/1 -> Mux3/5  "vy"
  Mux3/1 -> Out1/1
  Constant16/1 -> Mux3/7  "FR"
  Constant18/1 -> Mux3/9  "RL"
  Constant17/1 -> Mux3/8  "FL"
  Constant10/1 -> Mux3/1  "rotx"
  Constant15/1 -> Mux3/6  "vz"
  Constant13/1 -> Mux3/4  "vx"

== system RL_tcp_2021b/Evaluate actions/Subsystem1 ==
  0~1 : Inport
  Add : Sum  Inputs=+-
  Constant2 : Constant  Value=0.5
  Gain : Gain  Gain=2
  -1~1 : Outport
  wires:
  Gain/1 -> -1~1/1  "-1~1"
  Add/1 -> Gain/1
  Constant2/1 -> Add/2
  0~1/1 -> Add/1

== system RL_tcp_2021b/Reward/NN denorm ==
  In1 : Inport
  0~1to-1~1s : Subsystem  Commented=through
  Add : Sum
  Constant : Constant  Value=y_norm_min(4)  SampleTime=Ts
  Gain : Gain  Gain=y_norm_range(4)
  Out1 : Outport
  wires:
  Constant/1 -> Add/2
  Add/1 -> Out1/1
  Gain/1 -> Add/1
  In1/1 -> 0~1to-1~1s/1(In1)
  0~1to-1~1s/1(Out1) -> Gain/1

== system RL_tcp_2021b/Reward/Subsystem ==
  u : Inport
  AND : Logic  AllPortsSameDT=off  OutDataTypeStr=boolean
  AND1 : Logic  AllPortsSameDT=off  OutDataTypeStr=boolean
  AND2 : Logic  Operator=OR  AllPortsSameDT=off  OutDataTypeStr=boolean
  Compare To Constant : simulink/Logic and Bit Operations/Compare To Constant  relop=<=  const=0.2  OutDataTypeStr=boolean
  Compare To Constant1 : simulink/Logic and Bit Operations/Compare To Constant  relop=>=  const=0.8  OutDataTypeStr=boolean
  Compare To Constant2 : simulink/Logic and Bit Operations/Compare To Constant  relop=>=  const=0.8  OutDataTypeStr=boolean
  Compare To Constant3 : simulink/Logic and Bit Operations/Compare To Constant  relop=<=  const=0.2  OutDataTypeStr=boolean
  Demux : Demux
  Terminator : Terminator
  Terminator1 : Terminator
  Out1 : Outport
  wires:
  AND/1 -> AND2/1
  Compare To Constant/1 -> AND/1
  Demux/1 -> Compare To Constant1/1, Compare To Constant/1  "b1"
  Demux/3 -> Compare To Constant2/1, Compare To Constant3/1  "b2"
  Compare To Constant3/1 -> AND/2
  Demux/4 -> Terminator/1
  AND2/1 -> Out1/1
  Demux/2 -> Terminator1/1
  u/1 -> Demux/1
  Compare To Constant1/1 -> AND1/1
  Compare To Constant2/1 -> AND1/2
  AND1/1 -> AND2/2

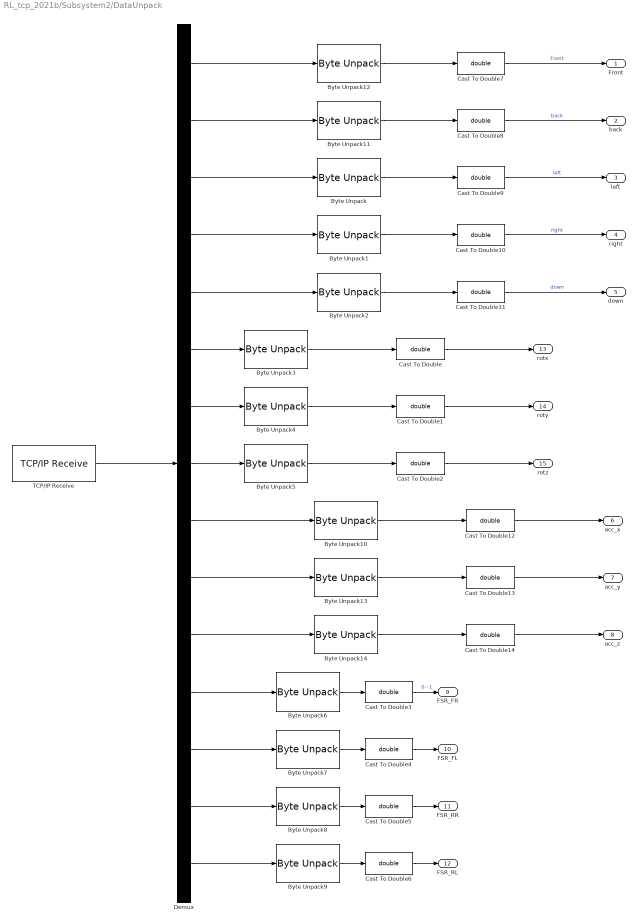
== system RL_tcp_2021b/Subsystem2/DataUnpack ==
  Byte Unpack{,1..14} (15 alike) : svdutilitieslib/Byte Unpack  dimensions={[1]}  datatypes={'single'}  byteAlign=1  blockPlatform=arduinoert
      settings: SourceProductBaseCode=ANDROID,ARDUINO,ML_ARDUINO,ECCORTEXA,ECCORTEXR,SC_BEAGLEBONE_BLUE,EC_FREEDOM_BOARD,EC_FRDM_K64F,INTEL_BLOCKSET,MICROBIT,NUCLEO,NVIDIA,PX4AUTOPILOTS,RASPPIIO,STMICRODIS,TIC2000,XILINX_BLOCKSET
  Cast To Double{,1..14} (15 alike) : DataTypeConversion  OutDataTypeStr=double
  Demux : Demux  Outputs=15
  TCP/IP Receive : instrumentlib/TCP//IP Receive  Priority=2  Host=192.168.0.103  Port=6666  DataSize=[60, 1 ]  DataType=uint8  ASCIIFormatting=%f  Terminator=LF  CustomTerminator=10  ByteOrder=big-endian  EnableBlockingMode=on  Timeout=1  SampleTime=Ts  SimulateUsing=Interpreted execution
  Front : Outport
  back : Outport  Port=2
  left : Outport  Port=3
  right : Outport  Port=4
  down : Outport  Port=5
  acc_x : Outport  Port=6
  acc_y : Outport  Port=7
  acc_z : Outport  Port=8
  FSR_FR : Outport  Port=9
  FSR_FL : Outport  Port=10
  FSR_RR : Outport  Port=11
  FSR_RL : Outport  Port=12
  rotx : Outport  Port=13
  roty : Outport  Port=14
  rotz : Outport  Port=15
  wires:
  Byte Unpack7/1 -> Cast To Double4/1
  Byte Unpack12/1 -> Cast To Double7/1
  Demux/5 -> Byte Unpack2/1
  Byte Unpack/1 -> Cast To Double9/1
  Byte Unpack6/1 -> Cast To Double3/1
  Demux/1 -> Byte Unpack12/1
  Demux/8 -> Byte Unpack5/1
  Demux/7 -> Byte Unpack4/1
  TCP/IP Receive/1 -> Demux/1
  Demux/3 -> Byte Unpack/1
  Demux/4 -> Byte Unpack1/1
  Byte Unpack4/1 -> Cast To Double1/1
  Byte Unpack8/1 -> Cast To Double5/1
  Demux/6 -> Byte Unpack3/1
  Byte Unpack2/1 -> Cast To Double11/1
  Demux/2 -> Byte Unpack11/1
  Byte Unpack5/1 -> Cast To Double2/1
  Byte Unpack9/1 -> Cast To Double6/1
  Byte Unpack1/1 -> Cast To Double10/1
  Byte Unpack3/1 -> Cast To Double/1
  Byte Unpack11/1 -> Cast To Double8/1
  Cast To Double3/1 -> FSR_FR/1  "0~1"
  Cast To Double4/1 -> FSR_FL/1
  Cast To Double5/1 -> FSR_RR/1
  Cast To Double6/1 -> FSR_RL/1
  Cast To Double/1 -> rotx/1
  Cast To Double2/1 -> rotz/1
  Cast To Double1/1 -> roty/1
  Cast To Double7/1 -> Front/1  "Front"
  Cast To Double8/1 -> back/1  "back"
  Cast To Double9/1 -> left/1  "left"
  Cast To Double10/1 -> right/1  "right"
  Cast To Double11/1 -> down/1  "down"
  Demux/15 -> Byte Unpack9/1
  Demux/14 -> Byte Unpack8/1
  Demux/13 -> Byte Unpack7/1
  Demux/12 -> Byte Unpack6/1
  Cast To Double14/1 -> acc_z/1
  Byte Unpack10/1 -> Cast To Double12/1
  Cast To Double12/1 -> acc_x/1
  Cast To Double13/1 -> acc_y/1
  Byte Unpack13/1 -> Cast To Double13/1
  Byte Unpack14/1 -> Cast To Double14/1
  Demux/9 -> Byte Unpack10/1
  Demux/10 -> Byte Unpack13/1
  Demux/11 -> Byte Unpack14/1

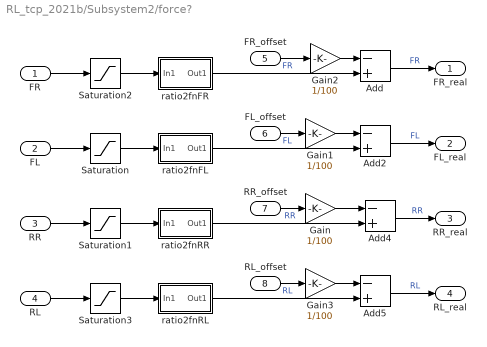
== system RL_tcp_2021b/Subsystem2/force? ==
  FR : Inport
  FL : Inport  Port=2
  RR : Inport  Port=3
  RL : Inport  Port=4
  FR_offset : Inport  Port=5
  FL_offset : Inport  Port=6
  RR_offset : Inport  Port=7
  RL_offset : Inport  Port=8
  Add{,2,4..5} (4 alike) : Sum  Inputs=-+
  Gain{,1..3} (4 alike) : Gain  Gain=1/100
  Saturation : Saturate  UpperLimit=0.99  LowerLimit=0.01
  Saturation1 : Saturate  UpperLimit=0.99  LowerLimit=0.01
  Saturation2 : Saturate  UpperLimit=0.99  LowerLimit=0.01
  Saturation3 : Saturate  UpperLimit=0.999  LowerLimit=0.01
  ratio2fnFL : Subsystem
  ratio2fnFR : Subsystem
  ratio2fnRL : Subsystem
  ratio2fnRR : Subsystem
  FR_real : Outport
  FL_real : Outport  Port=2
  RR_real : Outport  Port=3
  RL_real : Outport  Port=4
  wires:
  Saturation3/1 -> ratio2fnRL/1(In1)
  Add2/1 -> FL_real/1  "FL"
  ratio2fnRR/1(Out1) -> Add4/2  "RR"
  ratio2fnFR/1(Out1) -> Add/2  "FR"
  Saturation2/1 -> ratio2fnFR/1(In1)
  FL_offset/1 -> Gain1/1
  RL/1 -> Saturation3/1
  Saturation/1 -> ratio2fnFL/1(In1)
  ratio2fnFL/1(Out1) -> Add2/2  "FL"
  FL/1 -> Saturation/1
  FR/1 -> Saturation2/1
  Saturation1/1 -> ratio2fnRR/1(In1)
  ratio2fnRL/1(Out1) -> Add5/2  "RL"
  RR/1 -> Saturation1/1
  Add4/1 -> RR_real/1  "RR"
  RR_offset/1 -> Gain/1
  Add/1 -> FR_real/1  "FR"
  RL_offset/1 -> Gain3/1
  FR_offset/1 -> Gain2/1
  Add5/1 -> RL_real/1  "RL"
  Gain/1 -> Add4/1
  Gain1/1 -> Add2/1
  Gain2/1 -> Add/1
  Gain3/1 -> Add5/1

== system RL_tcp_2021b/Subsystem2/rot_cal ==
  rotx_offset : Inport
  roty_offset : Inport  Port=2
  rotz_offset : Inport  Port=3
  euler : Inport  Port=4
  Add7 : Sum  Inputs=+-
  Add8 : Sum  Inputs=+-
  Add9 : Sum  Inputs=+-
  Demux1 : Demux  Outputs=3
  Subsystem : Subsystem
  Subsystem1 : Subsystem
  Subsystem2 : Subsystem
  rotz : Outport
  rotx : Outport  Port=2
  roty : Outport  Port=3
  wires:
  euler/1 -> Demux1/1  "rot"
  Add7/1 -> rotz/1  "rotz"
  rotz_offset/1 -> Add7/2
  Demux1/1 -> Subsystem2/1(rotx_raw)  "rotx"
  Demux1/2 -> Subsystem1/1(roty_raw)  "roty"
  Demux1/3 -> Subsystem/1(rotz_raw)  "rotz"
  roty_offset/1 -> Add8/2
  rotx_offset/1 -> Add9/2
  Add9/1 -> rotx/1  "rotx"
  Add8/1 -> roty/1  "roty"
  Subsystem/1(rotz) -> Add7/1
  Subsystem1/1(roty) -> Add8/1
  Subsystem2/1(rotx) -> Add9/1

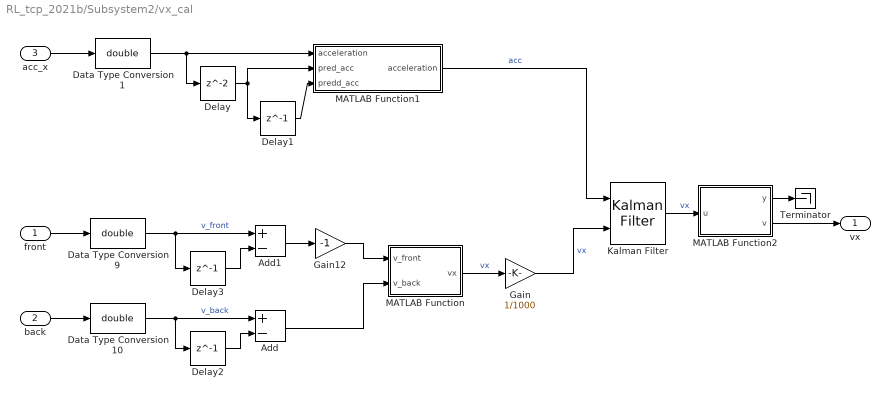
== system RL_tcp_2021b/Subsystem2/vx_cal ==
  front : Inport
  back : Inport  Port=2
  acc_x : Inport  Port=3
  Add : Sum  Inputs=+-
  Add1 : Sum  Inputs=+-
  Data Type Conversion1 : DataTypeConversion  OutDataTypeStr=double
  Data Type Conversion10 : DataTypeConversion  OutDataTypeStr=double
  Data Type Conversion9 : DataTypeConversion  OutDataTypeStr=double
  Delay : Delay  SampleTime=Ts
  Delay1 : Delay  DelayLength=1  SampleTime=Ts
  Delay2 : Delay  DelayLength=1  SampleTime=Ts
  Delay3 : Delay  DelayLength=1  InitialCondition=1500  SampleTime=Ts
  Gain : Gain  Gain=1/1000
  Gain12 : Gain  Gain=-1
  Kalman Filter : ctrlSharedLib/Kalman Filter  TimeDomain=Discrete-Time  UseCurrentEstimator=on  ModelSource=Individual A, B, C, D matrices  ModelSourceVariable=ss(0.95,1,1,0,1)  A=A  B=B  C=C  D=0  NumberOfStates=1  NumberOfInputs=1  NumberOfOutputs=1  InitialEstimateSource=Dialog  X0=[0;0]  P0=10  UseK=off  UseGH=off  NumberOfProcessNoiseInputs=1  G=1  TimeInvariantG=on  H=0  TimeInvariantH=on  Q=Q  TimeInvariantQ=on  R=R  TimeInvariantR=on  N=0  TimeInvariantN=on  AddInputPort=on  AddEnablePort=off  OutputEstimatedY=off  OutputP=off  Ts=Ts
  MATLAB Function : MATLAB Function  TreatAsAtomicUnit=on
  MATLAB Function1 : MATLAB Function  TreatAsAtomicUnit=on
  MATLAB Function2 : MATLAB Function  TreatAsAtomicUnit=on
  Terminator : Terminator
  vx : Outport
  wires:
  MATLAB Function/1(vx) -> Gain/1  "vx"
  Data Type Conversion9/1 -> Add1/1, Delay3/1  "v_front"
  Add1/1 -> Gain12/1
  front/1 -> Data Type Conversion9/1
  back/1 -> Data Type Conversion10/1
  Gain12/1 -> MATLAB Function/1(v_front)
  Kalman Filter/1 -> MATLAB Function2/1(u)  "vx"
  acc_x/1 -> Data Type Conversion1/1
  Delay/1 -> MATLAB Function1/2(pred_acc), Delay1/1
  Delay1/1 -> MATLAB Function1/3(predd_acc)
  Data Type Conversion10/1 -> Delay2/1, Add/1  "v_back"
  Delay2/1 -> Add/2
  Add/1 -> MATLAB Function/2(v_back)
  Delay3/1 -> Add1/2
  MATLAB Function1/1(acceleration) -> Kalman Filter/1  "acc"
  Gain/1 -> Kalman Filter/2  "vx"
  MATLAB Function2/1(y) -> Terminator/1
  MATLAB Function2/2(v) -> vx/1
  Data Type Conversion1/1 -> MATLAB Function1/1("acceleration "), Delay/1

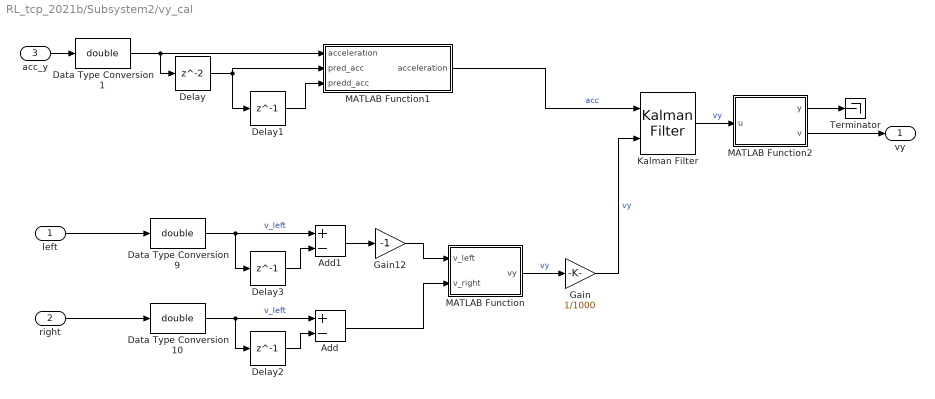
== system RL_tcp_2021b/Subsystem2/vy_cal ==
  left : Inport
  right : Inport  Port=2
  acc_y : Inport  Port=3
  Add : Sum  Inputs=+-
  Add1 : Sum  Inputs=+-
  Data Type Conversion1 : DataTypeConversion  OutDataTypeStr=double
  Data Type Conversion10 : DataTypeConversion  OutDataTypeStr=double
  Data Type Conversion9 : DataTypeConversion  OutDataTypeStr=double
  Delay : Delay  SampleTime=Ts
  Delay1 : Delay  DelayLength=1  SampleTime=Ts
  Delay2 : Delay  DelayLength=1  InitialCondition=600  SampleTime=Ts
  Delay3 : Delay  DelayLength=1  InitialCondition=200  SampleTime=Ts
  Gain : Gain  Gain=1/1000
  Gain12 : Gain  Gain=-1
  Kalman Filter : ctrlSharedLib/Kalman Filter  TimeDomain=Discrete-Time  UseCurrentEstimator=on  ModelSource=Individual A, B, C, D matrices  ModelSourceVariable=ss(0.95,1,1,0,1)  A=A  B=B  C=C  D=0  NumberOfStates=1  NumberOfInputs=1  NumberOfOutputs=1  InitialEstimateSource=Dialog  X0=[0;0]  P0=10  UseK=off  UseGH=off  NumberOfProcessNoiseInputs=1  G=1  TimeInvariantG=on  H=0  TimeInvariantH=on  Q=Q  TimeInvariantQ=on  R=R  TimeInvariantR=on  N=0  TimeInvariantN=on  AddInputPort=on  AddEnablePort=off  OutputEstimatedY=off  OutputP=off  Ts=Ts
  MATLAB Function : MATLAB Function  TreatAsAtomicUnit=on
  MATLAB Function1 : MATLAB Function  TreatAsAtomicUnit=on
  MATLAB Function2 : MATLAB Function  TreatAsAtomicUnit=on
  Terminator : Terminator
  vy : Outport
  wires:
  Delay1/1 -> MATLAB Function1/3(predd_acc)
  Delay/1 -> MATLAB Function1/2(pred_acc), Delay1/1
  acc_y/1 -> Data Type Conversion1/1
  MATLAB Function1/1(acceleration) -> Kalman Filter/1  "acc"
  Delay3/1 -> Add1/2
  Gain12/1 -> MATLAB Function/1(v_left)
  Data Type Conversion10/1 -> Delay2/1, Add/1  "v_left"
  right/1 -> Data Type Conversion10/1
  MATLAB Function/1(vy) -> Gain/1  "vy"
  left/1 -> Data Type Conversion9/1
  Data Type Conversion9/1 -> Add1/1, Delay3/1  "v_left"
  Gain/1 -> Kalman Filter/2  "vy"
  Delay2/1 -> Add/2
  Add/1 -> MATLAB Function/2(v_right)
  Add1/1 -> Gain12/1
  Data Type Conversion1/1 -> Delay/1, MATLAB Function1/1("acceleration ")
  Kalman Filter/1 -> MATLAB Function2/1(u)  "vy"
  MATLAB Function2/1(y) -> Terminator/1
  MATLAB Function2/2(v) -> vy/1

== system RL_tcp_2021b/Subsystem2/vy_cal1 ==
  down : Inport
  acc_z : Inport  Port=2
  Add1 : Sum  Inputs=+-
  Data Type Conversion1 : DataTypeConversion  OutDataTypeStr=double
  Data Type Conversion9 : DataTypeConversion  OutDataTypeStr=double
  Delay : Delay  SampleTime=Ts
  Delay1 : Delay  DelayLength=1  SampleTime=Ts
  Delay3 : Delay  DelayLength=1  SampleTime=Ts
  Gain : Gain  Gain=1/1000
  Gain12 : Gain  Gain=-1
  Kalman Filter : ctrlSharedLib/Kalman Filter  TimeDomain=Discrete-Time  UseCurrentEstimator=on  ModelSource=Individual A, B, C, D matrices  ModelSourceVariable=ss(0.95,1,1,0,1)  A=A  B=B  C=C  D=0  NumberOfStates=1  NumberOfInputs=1  NumberOfOutputs=1  InitialEstimateSource=Dialog  X0=[0;0]  P0=10  UseK=off  UseGH=off  NumberOfProcessNoiseInputs=1  G=1  TimeInvariantG=on  H=0  TimeInvariantH=on  Q=Q  TimeInvariantQ=on  R=R  TimeInvariantR=on  N=0  TimeInvariantN=on  AddInputPort=on  AddEnablePort=off  OutputEstimatedY=off  OutputP=off  Ts=Ts
  MATLAB Function : MATLAB Function  TreatAsAtomicUnit=on
  MATLAB Function1 : MATLAB Function  TreatAsAtomicUnit=on
  MATLAB Function2 : MATLAB Function  TreatAsAtomicUnit=on
  Terminator : Terminator
  vz : Outport
  wires:
  Delay1/1 -> MATLAB Function1/3(predd_acc)
  Delay/1 -> MATLAB Function1/2(pred_acc), Delay1/1
  acc_z/1 -> Data Type Conversion1/1
  MATLAB Function1/1(acceleration) -> Kalman Filter/1  "acc"
  Delay3/1 -> Add1/2
  Gain12/1 -> MATLAB Function/1(v_down)
  MATLAB Function/1(vz) -> Gain/1  "vz"
  down/1 -> Data Type Conversion9/1
  Data Type Conversion9/1 -> Add1/1, Delay3/1
  Gain/1 -> Kalman Filter/2  "vz"
  Add1/1 -> Gain12/1  "v_down"
  Data Type Conversion1/1 -> Delay/1, MATLAB Function1/1("acceleration ")
  Kalman Filter/1 -> MATLAB Function2/1(u)  "vz"
  MATLAB Function2/2(v) -> vz/1
  MATLAB Function2/1(y) -> Terminator/1

== system RL_tcp_2021b/Reward/NN denorm/0~1to-1~1s ==
  In1 : Inport
  Add : Sum  Inputs=+-
  Constant : Constant  Value=0.5  SampleTime=Ts
  Gain : Gain  Gain=2
  Out1 : Outport
  wires:
  Gain/1 -> Out1/1
  Constant/1 -> Add/2
  Add/1 -> Gain/1
  In1/1 -> Add/1

== system RL_tcp_2021b/Subsystem2/force?/ratio2fnFL ==
  In1 : Inport
  Add : Sum  Inputs=+-
  Add4 : Sum
  Constant : Constant  SampleTime=-1
  Constant4 : Constant  Value=fitresultpowertwoFL.a  SampleTime=-1
  Constant5 : Constant  Value=fitresultpowertwoFL.c  SampleTime=-1
  Constant6 : Constant  Value=fitresultpowertwoFL.b  SampleTime=-1
  Divide : Product  Inputs=/*
  Divide4 : Product  Inputs=**
  Gain : Gain  Gain=1567
  Power : Math  Operator=pow  SaturateOnIntegerOverflow=on
  Out1 : Outport
  wires:
  Constant/1 -> Add/1
  Add/1 -> Divide/1
  In1/1 -> Gain/1, Add/2
  Divide/1 -> Power/1  "Ohm"
  Divide4/1 -> Add4/2
  Constant5/1 -> Add4/1
  Power/1 -> Divide4/2
  Constant6/1 -> Power/2
  Constant4/1 -> Divide4/1
  Add4/1 -> Out1/1  "N"
  Gain/1 -> Divide/2

== system RL_tcp_2021b/Subsystem2/force?/ratio2fnFR ==
  In1 : Inport
  Add : Sum  Inputs=+-
  Add4 : Sum
  Constant : Constant  SampleTime=-1
  Constant4 : Constant  Value=fitresultpowertwoFR.a  SampleTime=-1
  Constant5 : Constant  Value=fitresultpowertwoFR.c  SampleTime=-1
  Constant6 : Constant  Value=fitresultpowertwoFR.b  SampleTime=-1
  Divide : Product  Inputs=/*
  Divide4 : Product  Inputs=**
  Gain : Gain  Gain=1567
  Power : Math  Operator=pow  SaturateOnIntegerOverflow=on
  Out1 : Outport
  wires:
  Add4/1 -> Out1/1  "N"
  Constant6/1 -> Power/2
  Constant/1 -> Add/1
  In1/1 -> Gain/1, Add/2
  Divide/1 -> Power/1  "ohm"
  Constant5/1 -> Add4/1
  Divide4/1 -> Add4/2
  Add/1 -> Divide/1
  Power/1 -> Divide4/2
  Constant4/1 -> Divide4/1
  Gain/1 -> Divide/2

== system RL_tcp_2021b/Subsystem2/force?/ratio2fnRL ==
  In1 : Inport
  Add3 : Sum  Inputs=+-
  Add7 : Sum
  Constant13 : Constant  Value=fitresultpowertwoRL.a  SampleTime=-1
  Constant14 : Constant  Value=fitresultpowertwoRL.c  SampleTime=-1
  Constant15 : Constant  Value=fitresultpowertwoRL.b  SampleTime=-1
  Constant3 : Constant  SampleTime=-1
  Divide3 : Product  Inputs=/*
  Divide7 : Product  Inputs=**
  Gain3 : Gain  Gain=1567
  Power3 : Math  Operator=pow  SaturateOnIntegerOverflow=on
  Out1 : Outport
  wires:
  Add7/1 -> Out1/1  "N"
  In1/1 -> Gain3/1, Add3/2
  Constant13/1 -> Divide7/1
  Add3/1 -> Divide3/1
  Divide7/1 -> Add7/2
  Constant14/1 -> Add7/1
  Constant3/1 -> Add3/1
  Constant15/1 -> Power3/2
  Power3/1 -> Divide7/2
  Divide3/1 -> Power3/1  "Ohm"
  Gain3/1 -> Divide3/2

== system RL_tcp_2021b/Subsystem2/force?/ratio2fnRR ==
  In1 : Inport
  Add2 : Sum  Inputs=+-
  Add6 : Sum
  Constant10 : Constant  Value=fitresultpowertwoRR.a  SampleTime=-1
  Constant11 : Constant  Value=fitresultpowertwoRR.c  SampleTime=-1
  Constant12 : Constant  Value=fitresultpowertwoRR.b  SampleTime=-1
  Constant2 : Constant  SampleTime=-1
  Divide2 : Product  Inputs=/*
  Divide6 : Product  Inputs=**
  Gain2 : Gain  Gain=1567
  Power2 : Math  Operator=pow  SaturateOnIntegerOverflow=on
  Out1 : Outport
  wires:
  In1/1 -> Gain2/1, Add2/2
  Divide6/1 -> Add6/2
  Power2/1 -> Divide6/2
  Constant2/1 -> Add2/1
  Constant10/1 -> Divide6/1
  Add2/1 -> Divide2/1
  Constant12/1 -> Power2/2
  Divide2/1 -> Power2/1  "Ohm"
  Constant11/1 -> Add6/1
  Add6/1 -> Out1/1  "N"
  Gain2/1 -> Divide2/2

== system RL_tcp_2021b/Subsystem2/rot_cal/Subsystem ==
  rotz_raw : Inport
  Abs : Abs
  Delay : Delay  DelayLength=1
  Subtract : Sum  Inputs=-+
  Switch : Switch  Criteria=u2 > Threshold  Threshold=0.2
  rotz : Outport
  wires:
  rotz_raw/1 -> Switch/3, Subtract/2
  Delay/1 -> Switch/1, Subtract/1
  Abs/1 -> Switch/2
  Subtract/1 -> Abs/1
  Switch/1 -> Delay/1, rotz/1

== system RL_tcp_2021b/Subsystem2/rot_cal/Subsystem1 ==
  roty_raw : Inport
  Abs : Abs
  Delay : Delay  DelayLength=1
  Subtract : Sum  Inputs=-+
  Switch : Switch  Criteria=u2 > Threshold  Threshold=0.2
  roty : Outport
  wires:
  roty_raw/1 -> Switch/3, Subtract/2
  Delay/1 -> Switch/1, Subtract/1
  Abs/1 -> Switch/2
  Subtract/1 -> Abs/1
  Switch/1 -> Delay/1, roty/1

== system RL_tcp_2021b/Subsystem2/rot_cal/Subsystem2 ==
  rotx_raw : Inport
  Abs : Abs
  Delay : Delay  DelayLength=1
  Subtract : Sum  Inputs=-+
  Switch : Switch  Criteria=u2 > Threshold  Threshold=0.2
  rotx : Outport
  wires:
  rotx_raw/1 -> Switch/3, Subtract/2
  Delay/1 -> Switch/1, Subtract/1
  Abs/1 -> Switch/2
  Subtract/1 -> Abs/1
  Switch/1 -> Delay/1, rotx/1

== matlab function RL_tcp_2021b/Subsystem2/vx_cal/MATLAB Function1 ==
  data: acceleration input; acceleration output; pred_acc input; predd_acc input
function acceleration = fcn(acceleration,pred_acc,predd_acc)
    if abs(acceleration) < 0.1
        acceleration = 0;
    end
    
    if abs(acceleration) > 10
        acceleration = (pred_acc+predd_acc)/2;
    end
end

== matlab function RL_tcp_2021b/Subsystem2/vy_cal/MATLAB Function ==
  data: v_left input; vy output; v_right input
function vy = fcn(v_left, v_right)

if abs(v_left) >= 20 && abs(v_right) < 20
    vy = v_right;
elseif abs(v_right) >= 20 && abs(v_left) < 20
    vy = v_left;
else
    vy = (v_right + v_left)/2;
end

== matlab function RL_tcp_2021b/Subsystem2/vx_cal/MATLAB Function2 ==
  data: u input; y output; v output
function [y, v] = fcn(u)

y = u(1);
v = u(2);

== matlab function RL_tcp_2021b/Subsystem2/vy_cal/MATLAB Function1 ==
  data: acceleration input; acceleration output; pred_acc input; predd_acc input
function acceleration = fcn(acceleration,pred_acc,predd_acc)
    if abs(acceleration) < 0.1
        acceleration = 0;
    end
    
    if abs(acceleration) > 10
        acceleration = (pred_acc+predd_acc)/2;
    end
end

== matlab function RL_tcp_2021b/Subsystem2/vy_cal1/MATLAB Function ==
  data: v_down input; vz output
function vz = fcn(v_down)

if v_down >= 20 
    vz = 20;
elseif v_down <= -20
    vz = -20;
else
    vz = v_down;
end

== matlab function RL_tcp_2021b/Subsystem2/vy_cal1/MATLAB Function1 ==
  data: acceleration input; acceleration output; pred_acc input; predd_acc input
function acceleration = fcn(acceleration,pred_acc,predd_acc)
    if abs(acceleration) < 0.1
        acceleration = 0;
    end
    
    if abs(acceleration) > 10
        acceleration = (pred_acc+predd_acc)/2;
    end
end

== matlab function RL_tcp_2021b/Subsystem2/vy_cal/MATLAB Function2 ==
  data: u input; y output; v output
function [y, v] = fcn(u)

y = u(1);
v = u(2);

== matlab function RL_tcp_2021b/Subsystem2/vy_cal1/MATLAB Function2 ==
  data: u input; y output; v output
function [y, v] = fcn(u)

y = u(1);
v = u(2);

== matlab function RL_tcp_2021b/evaluateActions/MATLAB Function1 ==
  data: action1 output double; meanAndStd input
function action1 = evaluatePolicy(meanAndStd)
%#codegen

% Reinforcement Learning Toolbox
% Generated on: 26-Sep-2023 11:56:57

numAction = 4;
actionMean = meanAndStd(1:numAction);


% Ranges of all action dimensiosn are bounded.
action1 = tanh(actionMean).*0.5 + 0.5;
end

== matlab function RL_tcp_2021b/Subsystem2/vx_cal/MATLAB Function ==
  data: v_front input; vx output; v_back input
function vx = fcn(v_front, v_back)

if abs(v_front) >= 20 && abs(v_back) < 20
    vx = v_back;
elseif abs(v_back) >= 20 && abs(v_front) < 20
    vx = v_front;
else
    vx = (v_back + v_front)/2;
end

== matlab function RL_tcp_2021b/evaluateActions/MATLAB Function2 ==
  data: action1 output double; data input
function action1 = evaluateActions(data)
numAction = 12;

actionMean = data(1:numAction);
actionStd = data(numAction+1:end);

% Sample action from mean and standard deviation
action1 = actionMean + actionStd .* randn(size(actionMean),'like',actionMean);

action1 = reshape(action1,[],1);

% Ranges of all action dimensiosn are bounded.
action1 = tanh(action1)*0.5 + 0.5;
% action1 = reshape(action1,[12   1]);

== matlab function RL_tcp_2021b/GoldenGait/FL ==
  data: alpha_r input; alpha_A output; alpha_b input; z_l input; alpha_B output; alpha_C output
function [alpha_A, alpha_B, alpha_C]= fcn(alpha_r, alpha_b, z_l)

L_disk = 0.02944;% Disk side length (m)
R_spool = 0.021;
R_w = L_disk/sqrt(3);

alpha_A = -(-R_w*alpha_b*cos(-alpha_r)+z_l)/R_spool;
alpha_B = -(-R_w*alpha_b*cos(-alpha_r+2*pi/3)+z_l)/R_spool;
alpha_C = -(-R_w*alpha_b*cos(-alpha_r+4*pi/3)+z_l)/R_spool;

== matlab function RL_tcp_2021b/GoldenGait/FR ==
  data: alpha_r input; alpha_A output; alpha_b input; z_l input; alpha_B output; alpha_C output
function [alpha_A, alpha_B, alpha_C]= fcn(alpha_r, alpha_b, z_l)

L_disk = 0.02944;% Disk side length (m)
R_spool = 0.021;
R_w = L_disk/sqrt(3);

alpha_A = -(-R_w*alpha_b*cos(-alpha_r)+z_l)/R_spool;
alpha_B = -(-R_w*alpha_b*cos(-alpha_r+2*pi/3)+z_l)/R_spool;
alpha_C = -(-R_w*alpha_b*cos(-alpha_r+4*pi/3)+z_l)/R_spool;

== matlab function RL_tcp_2021b/GoldenGait/RL ==
  data: alpha_r input; alpha_A output; alpha_b input; z_l input; alpha_B output; alpha_C output
function [alpha_A, alpha_B, alpha_C]= fcn(alpha_r, alpha_b, z_l)

L_disk = 0.02944;% Disk side length (m)
R_spool = 0.021;
R_w = L_disk/sqrt(3);

alpha_A = -(-R_w*alpha_b*cos(-alpha_r)+z_l)/R_spool;
alpha_B = -(-R_w*alpha_b*cos(-alpha_r+2*pi/3)+z_l)/R_spool;
alpha_C = -(-R_w*alpha_b*cos(-alpha_r+4*pi/3)+z_l)/R_spool;

== matlab function RL_tcp_2021b/GoldenGait/RR ==
  data: alpha_r input; alpha_A output; alpha_b input; z_l input; alpha_B output; alpha_C output
function [alpha_A, alpha_B, alpha_C]= fcn(alpha_r, alpha_b, z_l)

L_disk = 0.02944;% Disk side length (m)
R_spool = 0.021;
R_w = L_disk/sqrt(3);

alpha_A = -(-R_w*alpha_b*cos(-alpha_r)+z_l)/R_spool;
alpha_B = -(-R_w*alpha_b*cos(-alpha_r+2*pi/3)+z_l)/R_spool;
alpha_C = -(-R_w*alpha_b*cos(-alpha_r+4*pi/3)+z_l)/R_spool;

== matlab function RL_tcp_2021b/Evaluate actions/FR ==
  data: alpha_r input; alpha_A output; alpha_b input; z_l input; alpha_B output; alpha_C output
function [alpha_A, alpha_B, alpha_C]= fcn(alpha_r, alpha_b, z_l)

L_disk = 0.02944;% Disk side length (m)
R_spool = 0.021;
R_w = L_disk/sqrt(3);

alpha_A = -(-R_w*alpha_b*cos(-alpha_r)+z_l)/R_spool;
alpha_B = -(-R_w*alpha_b*cos(-alpha_r+2*pi/3)+z_l)/R_spool;
alpha_C = -(-R_w*alpha_b*cos(-alpha_r+4*pi/3)+z_l)/R_spool;

== matlab function RL_tcp_2021b/Evaluate actions/FL ==
  data: alpha_r input; alpha_A output; alpha_b input; z_l input; alpha_B output; alpha_C output
function [alpha_A, alpha_B, alpha_C]= fcn(alpha_r, alpha_b, z_l)

L_disk = 0.02944;% Disk side length (m)
R_spool = 0.021;
R_w = L_disk/sqrt(3);

alpha_A = -(-R_w*alpha_b*cos(-alpha_r)+z_l)/R_spool;
alpha_B = -(-R_w*alpha_b*cos(-alpha_r+2*pi/3)+z_l)/R_spool;
alpha_C = -(-R_w*alpha_b*cos(-alpha_r+4*pi/3)+z_l)/R_spool;
